simulink model "mfb"  (R2020b)
settings: Solver=VariableStepAuto  StartTime=0.0  StopTime=10.0  RelTol=1e-3
settings Model: Creator=Rocksmithed  LastModifiedBy=Rocksmithed

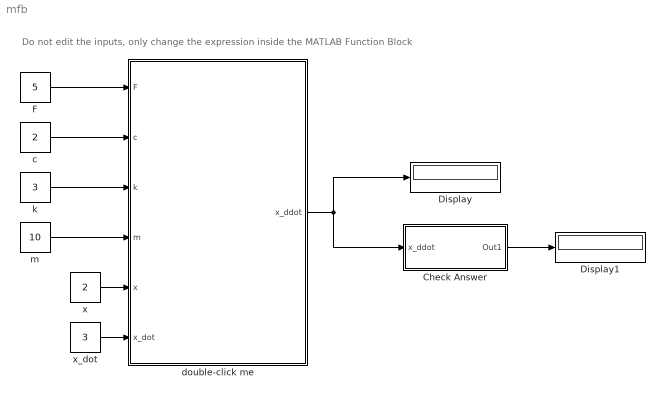
== system mfb ==
  note: Do not edit the inputs, only change the expression inside the MATLAB Function Block
  Check Answer : Subsystem
  Display : Display
  Display1 : Display
  F : Constant  Value=5
  c : Constant  Value=2
  double-click me : MATLAB Function  TreatAsAtomicUnit=on
  k : Constant  Value=3
  m : Constant  Value=10
  x : Constant  Value=2
  x_dot : Constant  Value=3
  wires:
  F/1 -> double-click me/1(F)
  c/1 -> double-click me/2(c)
  k/1 -> double-click me/3(k)
  m/1 -> double-click me/4(m)
  x/1 -> double-click me/5(x)
  x_dot/1 -> double-click me/6(x_dot)
  double-click me/1(x_ddot) -> Check Answer/1(x_ddot), Display/1
  Check Answer/1(Out1) -> Display1/1

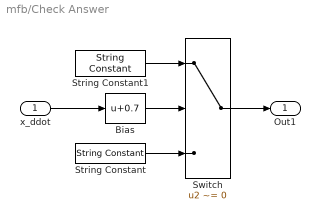
== system mfb/Check Answer ==
  x_ddot : Inport
  Bias : Bias  Bias=0.7
  String Constant : StringConstant  String="\"Correct\""
  String Constant1 : StringConstant  String="\"Incorrect\""
  Switch : Switch  Criteria=u2 ~= 0
  Out1 : Outport
  wires:
  x_ddot/1 -> Bias/1
  Bias/1 -> Switch/2
  Switch/1 -> Out1/1
  String Constant/1 -> Switch/3
  String Constant1/1 -> Switch/1

== matlab function mfb/double-click me ==
  data: F input; x_ddot output; c input; k input; m input; x input; x_dot input
function x_ddot = fcn(F,c,k,m,x,x_dot)

   % Replace NaN with your expression for x_ddot here in terms of the inputs
   x_ddot = NaN;
   
end
